simulink model "Rohrpendel"  (R2018a)
settings: Solver=VariableStepAuto  StartTime=0.0  StopTime=10.0  FixedStep=0.0001  MaxStep=0.01  RelTol=1e-3  EnableMultiTasking=on
model workspace (MATLAB code in the model file):
  | m1 = 0.1;    % kg
  | m2 = 0.08;  % kg
  | l = 0.3;         % m
  | g = 9.81;      % m/s^2
  | J = (m1 * l^2) /3;
  | k = 2;            % N/m
  | phi0 = pi/4;  % Achtelkreis
  | x0 = 0;          % m
settings Model: Creator=lohoefen  LastModifiedBy=manfred
settings DataIOCC: LimitDataPoints=on  SaveFormat=Array  SignalLoggingSaveFormat=ModelDataLogs
settings OptimizationCC: ExpressionDepthLimit=2147483647  LifeSpan=inf
settings DebuggingCC: UnderspecifiedInitializationDetection=Classic  MergeDetectMultiDrivingBlocksExec=none  SolverPrmCheckMsg=warning  FcnCallInpInsideContextMsg=warning  StateNameClashWarn=warning  SFUnexpectedBacktrackingDiag=warning  SFNoUnconditionalDefaultTransitionDiag=warning  SFExecutionAtInitializationDiag=none
settings HardwareCC: ProdBitPerPointer=32  ProdBitPerSizeT=32  ProdBitPerPtrDiffT=32  ProdLargestAtomicFloat=None  ProdIntDivRoundTo=Undefined  ProdEndianess=Unspecified  ProdWordSize=32  ProdHWDeviceType=32-bit Generic
settings ModelReferenceCC: PropagateSignalLabelsOutOfModel=off
settings CodeAppCC: StateflowObjectComments=on
settings GRTTargetCC: TargetLangStandard=C89/C90 (ANSI)  CombineOutputUpdateFcns=off  GRTInterface=on
settings ConfigComp: CovMetricSettings=dw  CovHtmlReporting=on  CovSaveCumulativeToWorkspaceVar=on  CovSaveSingleToWorkspaceVar=on  CovExternalEMLEnable=off

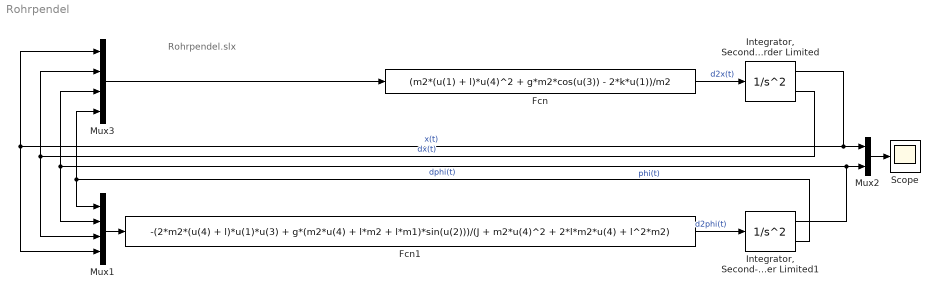
== system Rohrpendel ==
  note: Rohrpendel.slx
  Fcn : Fcn  Expr=(m2*(u(1) + l)*u(4)^2 + g*m2*cos(u(3)) - 2*k*u(1))/m2
  Fcn1 : Fcn  Expr=-(2*m2*(u(4) + l)*u(1)*u(3) + g*(m2*u(4) + l*m2 + l*m1)*sin(u(2)))/(J + m2*u(4)^2 + 2*l*m2*u(4) + l^2*m2)
  "Integrator, Second-Order Limited" : SecondOrderIntegrator  ICX=x0  LimitX=on  UpperLimitX=1  LowerLimitX=0  LimitDXDT=on
  "Integrator, Second-Order Limited1" : SecondOrderIntegrator  ICX=phi0  LimitX=on  UpperLimitX=1  LowerLimitX=0  LimitDXDT=on
  Mux1 : Mux
  Mux2 : Mux  Inputs=2
  Mux3 : Mux
  Scope : Scope
  wires:
  Fcn/1 -> "Integrator, Second-Order Limited"/1  "d2x(t)"
  Mux3/1 -> Fcn/1
  "Integrator, Second-Order Limited"/2 -> Mux3/2, Mux1/3  "dx(t)"
  Fcn1/1 -> "Integrator, Second-Order Limited1"/1  "d2phi(t)"
  "Integrator, Second-Order Limited1"/2 -> Mux1/1, Mux3/4  "dphi(t)"
  Mux2/1 -> Scope/1
  Mux1/1 -> Fcn1/1
  "Integrator, Second-Order Limited"/1 -> Mux2/1, Mux1/4, Mux3/1  "x(t)"
  "Integrator, Second-Order Limited1"/1 -> Mux2/2, Mux3/3, Mux1/2  "phi(t)"
